simulink model "phase1"  (R2015b)
settings: Solver=VariableStepAuto  StartTime=0.0  StopTime=29  RelTol=1e-3
values from neighbouring files (symbols this model uses):
  w = sys_wheelchair()    [CG.m]    (also in event_ode.m; main.m; odefun.m = sys_wheelchair; odefun2.m = sys_wheelchair)
libraries: simulink x1
settings Model: Creator=erive  LastModifiedBy=erive

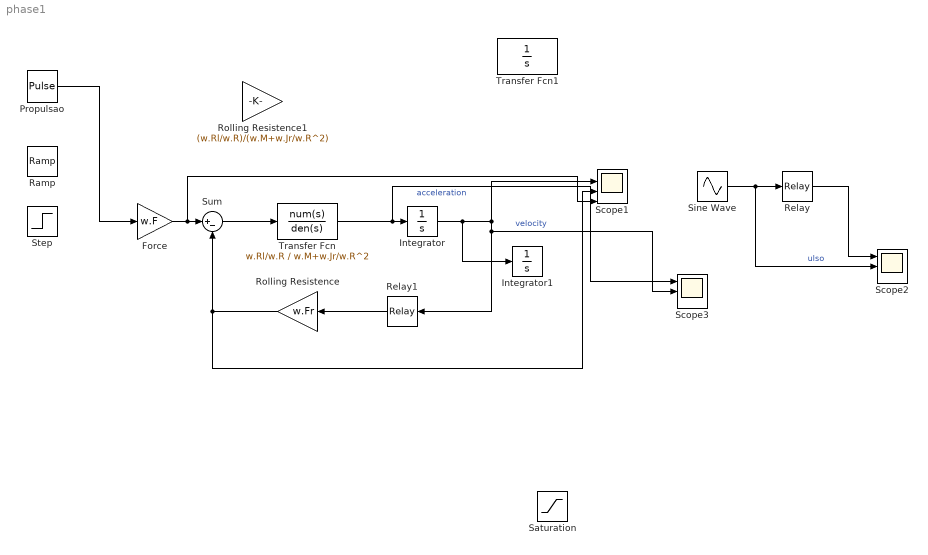
== system phase1 ==
  Force : Gain  Gain=w.F
  Integrator : Integrator
  Integrator1 : Integrator
  Propulsao : DiscretePulseGenerator  PulseType=Time based  Period=50  PulseWidth=25
  Ramp : simulink/Sources/Ramp  slope=1  start=0  X0=0
  Relay : Relay  OnSwitchValue=0.3  OffSwitchValue=-0.2  OutMin=-1  OutMax=1
  Relay1 : Relay  OnSwitchValue=0.5  OffSwitchValue=0  OutMin=-1  OutMax=1
  Rolling Resistence : Gain  Gain=w.Fr
  Rolling Resistence1 : Gain  Gain=(w.Rl/w.R)/(w.M+w.Jr/w.R^2)
  Saturation : Saturate
  Scope1 : Scope  NumInputPorts=4
  Scope2 : Scope  NumInputPorts=3
  Scope3 : Scope  NumInputPorts=3
  Sine Wave : Sin  Amplitude=4  Frequency=2*pi/20  SampleTime=0
  Step : Step  Time=0  SampleTime=0
  Sum : Sum  Inputs=|+-
  Transfer Fcn : TransferFcn  Numerator=w.Rl/w.R  Denominator=w.M+w.Jr/w.R^2
  Transfer Fcn1 : TransferFcn  Denominator=[1 0]
  wires:
  Rolling Resistence/1 -> Scope1/3, Sum/2
  Sum/1 -> Transfer Fcn/1
  Transfer Fcn/1 -> Scope3/1, Integrator/1  "acceleration"
  Integrator/1 -> Integrator1/1, Scope1/2, Scope3/2, Relay1/1  "velocity"
  Force/1 -> Scope1/4, Sum/1
  Propulsao/1 -> Force/1
  Relay/1 -> Scope2/1
  Sine Wave/1 -> Relay/1, Scope2/2  "ulso"
  Relay1/1 -> Rolling Resistence/1
